simulink model "lab2_sim"  (R2019b)
settings: Solver=ode45  StartTime=0.0  StopTime=Tfin  MaxStep=Tstep  RelTol=1e-3
values from neighbouring files (symbols this model uses):
  C = [1, 0, 0]    [lab2_prac.m]
  K = place(A, B , [-1, -2])    [lab2_prac.m]
  x0 = [0, 0, 0]    [lab2_prac.m]
undefined symbols (not defined in the file or in its folder): chua_fg, ga, mu_chua, ref_chua, u_chua
settings Model: Creator=user  LastModifiedBy=user

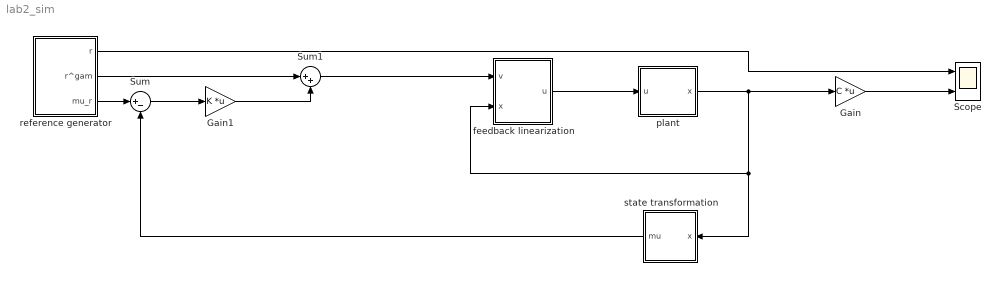
== system lab2_sim ==
  Gain : Gain  Gain=C  Multiplication=Matrix(K*u)
  Gain1 : Gain  Gain=K  Multiplication=Matrix(K*u)
  Scope : Scope  NumInputPorts=2
  Sum : Sum  Inputs=|+-
  Sum1 : Sum  Inputs=|++
  feedback linearization : Subsystem
  "plant " : Subsystem
  reference generator : Subsystem
  state transformation : Subsystem
  wires:
  "plant "/1(x) -> feedback linearization/2(x), state transformation/1(x), Gain/1
  feedback linearization/1(u) -> "plant "/1("u ")
  reference generator/3(mu_r) -> Sum/1
  state transformation/1(mu) -> Sum/2
  Sum/1 -> Gain1/1
  Gain1/1 -> Sum1/2
  Sum1/1 -> feedback linearization/1(v)
  reference generator/2(r^gam) -> Sum1/1
  Gain/1 -> Scope/2
  reference generator/1(r) -> Scope/1

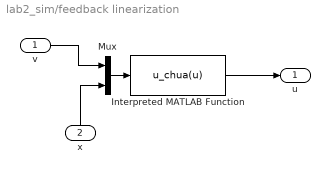
== system lab2_sim/feedback linearization ==
  v : Inport
  x : Inport  Port=2
  Interpreted MATLAB Function : MATLABFcn  MATLABFcn=u_chua(u)
  Mux : Mux  Inputs=2
  u : Outport  VectorParamsAs1DForOutWhenUnconnected=off
  wires:
  x/1 -> Mux/2
  Mux/1 -> Interpreted MATLAB Function/1
  v/1 -> Mux/1
  Interpreted MATLAB Function/1 -> u/1

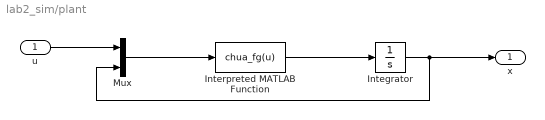
== system lab2_sim/plant  ==
  "u " : Inport
  Integrator : Integrator  InitialCondition=x0
  Interpreted MATLAB Function : MATLABFcn  MATLABFcn=chua_fg(u)
  Mux : Mux  Inputs=2
  x : Outport
  wires:
  Interpreted MATLAB Function/1 -> Integrator/1
  Mux/1 -> Interpreted MATLAB Function/1
  "u "/1 -> Mux/1
  Integrator/1 -> x/1, Mux/2

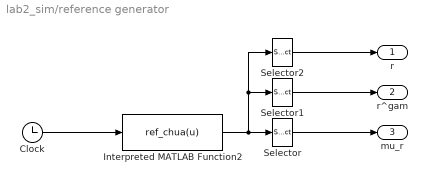
== system lab2_sim/reference generator ==
  Clock : Clock
  Interpreted MATLAB Function2 : MATLABFcn  MATLABFcn=ref_chua(u)
  Selector : Selector  InputPortWidth=ga+1  IndexOptions=Index vector (dialog)  Indices=1:ga  OutputSizes=1
  Selector1 : Selector  InputPortWidth=ga+1  IndexOptions=Index vector (dialog)  Indices=ga+1  OutputSizes=1
  Selector2 : Selector  InputPortWidth=ga+1  IndexOptions=Index vector (dialog)  Indices=1  OutputSizes=1
  r : Outport  VectorParamsAs1DForOutWhenUnconnected=off
  r^gam : Outport  Port=2  VectorParamsAs1DForOutWhenUnconnected=off
  mu_r : Outport  Port=3  VectorParamsAs1DForOutWhenUnconnected=off
  wires:
  Clock/1 -> Interpreted MATLAB Function2/1
  Selector1/1 -> r^gam/1
  Selector2/1 -> r/1
  Interpreted MATLAB Function2/1 -> Selector2/1, Selector1/1, Selector/1
  Selector/1 -> mu_r/1

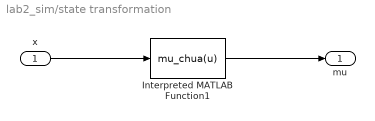
== system lab2_sim/state transformation ==
  x : Inport
  Interpreted MATLAB Function1 : MATLABFcn  MATLABFcn=mu_chua(u)
  mu : Outport  VectorParamsAs1DForOutWhenUnconnected=off
  wires:
  x/1 -> Interpreted MATLAB Function1/1
  Interpreted MATLAB Function1/1 -> mu/1
